simulink model "tempreture_control_5"  (R2021a)
settings: Solver=VariableStepAuto  StartTime=0.0  StopTime=10.0  RelTol=1e-3
settings Model: Creator=yasso  LastModifiedBy=yasso

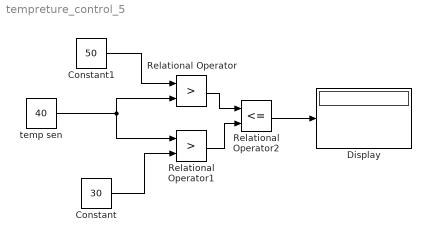
== system tempreture_control_5 ==
  Constant : Constant  Value=30
  Constant1 : Constant  Value=50
  Display : Display
  Relational Operator : RelationalOperator  Operator=>  OutDataTypeStr=boolean  RndMeth=Simplest
  Relational Operator1 : RelationalOperator  Operator=>  OutDataTypeStr=boolean  RndMeth=Simplest
  Relational Operator2 : RelationalOperator  Operator=<=  OutDataTypeStr=boolean  RndMeth=Simplest
  temp sen : Constant  Value=40
  wires:
  Constant/1 -> Relational Operator1/2
  Constant1/1 -> Relational Operator/1
  temp sen/1 -> Relational Operator1/1, Relational Operator/2
  Relational Operator/1 -> Relational Operator2/1
  Relational Operator1/1 -> Relational Operator2/2
  Relational Operator2/1 -> Display/1
